simulink model "Dynamic_Compensator_Linear"  (R2025b)
settings: Solver=VariableStepAuto  StartTime=0.0  StopTime=500  RelTol=1e-3
values from neighbouring files (symbols this model uses):
  AL = A-L*C    [fase1.m]
  BL = [Bu L]    [fase1.m]
  C = [1, 0, 0]    [fase1.m]
  CL = eye(size(A))    [fase1.m]
  DL = zeros(size(A,1),2)    [fase1.m]
  K = place(A, Bu, poles_SSF)    [fase1.m]
undefined symbols (not defined in the file or in its folder): A, B, xeq
settings Model: Creator=Rika  LastModifiedBy=Rika

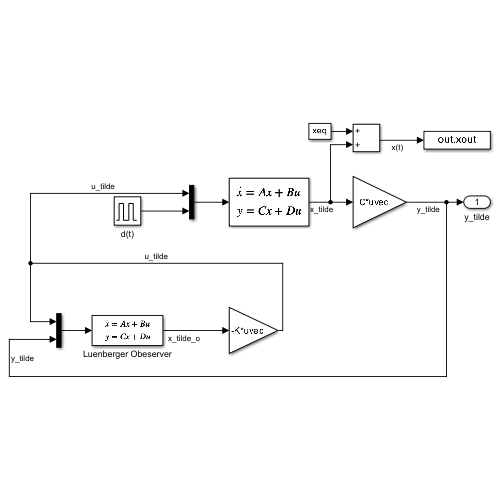
[thumbnail: Simulink's stored preview of the top-level diagram]
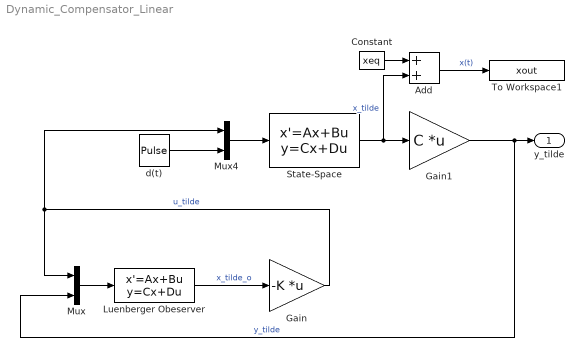
== system Dynamic_Compensator_Linear ==
  Add : Sum
  Constant : Constant  Value=xeq
  Gain : Gain  Gain=-K  Multiplication=Matrix(K*u) (u vector)
  Gain1 : Gain  Gain=C  Multiplication=Matrix(K*u) (u vector)
  Luenberger Obeserver : StateSpace  A=AL  B=BL  C=CL  D=DL  InitialCondition=0
  Mux : Mux  Inputs=2
  Mux4 : Mux  Inputs=2
  State-Space : StateSpace  A=A  B=B  C=eye(3)  D=zeros(3,2)  InitialCondition=0
  To Workspace1 : ToWorkspace  VariableName=xout  SaveFormat=Timeseries  SampleTime=-1
  d(t) : DiscretePulseGenerator  PulseType=Time based  Amplitude=10  Period=1000  PulseWidth=3  PhaseDelay=10
  y_tilde : Outport
  wires:
  Mux/1 -> Luenberger Obeserver/1
  Luenberger Obeserver/1 -> Gain/1  "x_tilde_o"
  Gain1/1 -> Mux/2, y_tilde/1  "y_tilde"
  Gain/1 -> Mux/1, Mux4/1  "u_tilde"
  d(t)/1 -> Mux4/2
  State-Space/1 -> Add/2, Gain1/1  "x_tilde"
  Mux4/1 -> State-Space/1
  Add/1 -> To Workspace1/1  "x(t)"
  Constant/1 -> Add/1
